simulink model "LR"  (R2021a)
settings: Solver=VariableStepAuto  StartTime=0.0  StopTime=10.0  RelTol=1e-3
libraries: commanapbnd3 x2
settings Model: Creator=Rubina  LastModifiedBy=Rubina

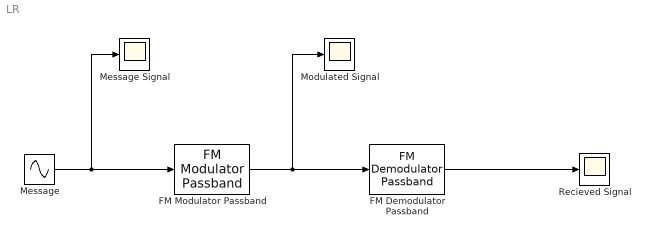
== system LR ==
  FM Demodulator Passband : commanapbnd3/FM Demodulator Passband  Fc=300  Ph=0  Kc=50  Ho=100
      settings: SourceProductBaseCode=CM
  FM Modulator Passband : commanapbnd3/FM Modulator Passband  Fc=300  Ph=0  Kc=50
      settings: SourceProductBaseCode=CM
  Message : Sin  Frequency=2*pi*5  SampleTime=1/8000
  Message Signal : Scope
  Modulated Signal : Scope
  Recieved Signal : Scope
  wires:
  Message/1 -> Message Signal/1, FM Modulator Passband/1
  FM Modulator Passband/1 -> Modulated Signal/1, FM Demodulator Passband/1
  FM Demodulator Passband/1 -> Recieved Signal/1
